simulink model "swingup_student_1"  (R2025b)
settings: Solver=VariableStepAuto  StartTime=0.0  StopTime=30  RelTol=1e-3
undefined symbols (not defined in the file): A, B, C, g, Jp_cm, K, kt, l, mp, mr, r, Rm
libraries: simulink_extras x4, simulink x4
settings Model: Creator=SURESH  LastModifiedBy=USER_NAME
settings RTWCC: GPUComputeCapability=3.5

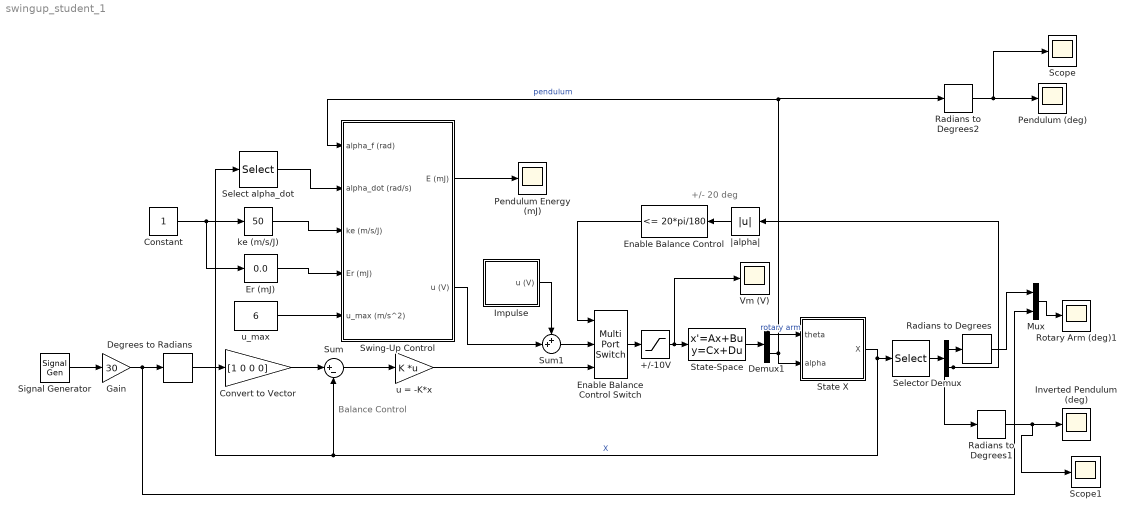
== system swingup_student_1 ==
  note: Balance Control
  note: +/- 20 deg
  +/-10V : Saturate  UpperLimit=10  LowerLimit=-10
  Constant : Constant
  Convert to Vector : Gain  Gain=[1 0 0 0]
  Degrees to Radians : simulink_extras/Transformations/Degrees to Radians
  Demux : Demux  Outputs=2
  Demux1 : Demux  Outputs=2
  Enable Balance Control : simulink/Logic and Bit Operations/Compare To Constant  relop=<=  const=20*pi/180  OutDataTypeStr=uint8  ZeroCross=off
  Enable Balance Control Switch : MultiPortSwitch  DataPortOrder=Zero-based contiguous  Inputs=2  zeroidx=on  SaturateOnIntegerOverflow=off  InputSameDT=off
  Er (mJ) : simulink/Math Operations/Slider Gain  gain=0.0  low=0  high=100
  Gain : Gain  Gain=30
  Impulse : Subsystem
  Inverted Pendulum (deg) : Scope
      settings: ActiveDisplayYMinimum=-5.36133  ActiveDisplayYMaximum=4.30664
  Mux : Mux  Inputs=2
  Pendulum (deg) : Scope
      settings: ActiveDisplayYMinimum=-3.91938  ActiveDisplayYMaximum=3.91995  DataLoggingVariableName=ScopeData2
  Pendulum Energy (mJ) : Scope
      settings: ActiveDisplayYMinimum=30.37049  ActiveDisplayYMaximum=30.37211  DataLoggingVariableName=ScopeData3
  Radians to Degrees : simulink_extras/Transformations/Radians to Degrees
  Radians to Degrees1 : simulink_extras/Transformations/Radians to Degrees
  Radians to Degrees2 : simulink_extras/Transformations/Radians to Degrees
  Rotary Arm (deg)1 : Scope
      settings: ActiveDisplayYMinimum=-42.00725544440256  ActiveDisplayYMaximum=43.502817755714887  DataLoggingVariableName=ScopeData4
  Scope : Scope
      settings: ActiveDisplayYMinimum=-8.16350735550788  ActiveDisplayYMaximum=8.1792601207942344  DataLoggingVariableName=ScopeData5
  Scope1 : Scope
      settings: ActiveDisplayYMinimum=-224.97803  ActiveDisplayYMaximum=224.80225  DataLoggingVariableName=ScopeData6
  Select alpha_dot : Selector  InputPortWidth=4  IndexOptions=Index vector (dialog)  Indices=[4]  OutputSizes=1
  Selector : Selector  InputPortWidth=4  IndexOptions=Index vector (dialog)  Indices=[1 2]  OutputSizes=1
  Signal Generator : SignalGenerator  WaveForm=square  Frequency=0.125
  State X : Subsystem
  State-Space : StateSpace  A=A  B=B  C=C  D=[0;0]  InitialCondition=0
  Sum : Sum  Inputs=|+-
  Sum1 : Sum  Inputs=++|
  Swing-Up Control : Subsystem
  Vm (V) : Scope
      settings: ActiveDisplayYMinimum=-4.30069  ActiveDisplayYMaximum=2.05211
  ke (m/s/J) : simulink/Math Operations/Slider Gain  gain=50  low=0  high=100
  u = -K*x : Gain  Gain=K  Multiplication=Matrix(K*u)
  u_max : Constant  Value=6
  |alpha| : Abs  SaturateOnIntegerOverflow=off
  wires:
  +/-10V/1 -> State-Space/1, Vm (V)/1
  Radians to Degrees/1 -> Mux/1
  Radians to Degrees2/1 -> Scope/1, Pendulum (deg)/1
  Er (mJ)/1 -> Swing-Up Control/4(Er (mJ))
  Convert to Vector/1 -> Sum/1
  Signal Generator/1 -> Gain/1
  Sum1/1 -> Enable Balance Control Switch/2
  Constant/1 -> Er (mJ)/1, ke (m/s/J)/1
  Sum/1 -> u = -K*x/1
  u_max/1 -> Swing-Up Control/5(u_max (m/s^2))
  Gain/1 -> Mux/2, Degrees to Radians/1
  Radians to Degrees1/1 -> Scope1/1, Inverted Pendulum (deg)/1
  Swing-Up Control/1(E (mJ)) -> Pendulum Energy (mJ)/1
  Mux/1 -> Rotary Arm (deg)1/1
  Swing-Up Control/2(u (V)) -> Sum1/2
  Enable Balance Control/1 -> Enable Balance Control Switch/1
  ke (m/s/J)/1 -> Swing-Up Control/3(ke (m/s/J))
  u = -K*x/1 -> Enable Balance Control Switch/3
  Demux/1 -> Radians to Degrees/1
  |alpha|/1 -> Enable Balance Control/1
  Select alpha_dot/1 -> Swing-Up Control/2(alpha_dot (rad/s))
  Degrees to Radians/1 -> Convert to Vector/1
  Enable Balance Control Switch/1 -> +/-10V/1
  Impulse/1(u (V)) -> Sum1/1
  Selector/1 -> Demux/1
  State X/1(X) -> Select alpha_dot/1, Sum/2, Selector/1  "X"
  Demux/2 -> Radians to Degrees1/1, |alpha|/1
  Demux1/1 -> State X/1(theta)  "rotary arm"
  State-Space/1 -> Demux1/1
  Demux1/2 -> Swing-Up Control/1(alpha_f (rad)), Radians to Degrees2/1, State X/2(alpha)  "pendulum"

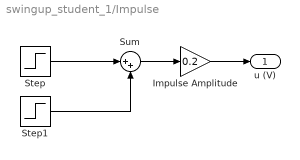
== system swingup_student_1/Impulse ==
  Impulse Amplitude : Gain  Gain=0.2
  Step : Step  SampleTime=0
  Step1 : Step  Time=1.1  After=-1  SampleTime=0
  Sum : Sum  Inputs=|++
  u (V) : Outport
  wires:
  Step1/1 -> Sum/2
  Step/1 -> Sum/1
  Sum/1 -> Impulse Amplitude/1
  Impulse Amplitude/1 -> u (V)/1

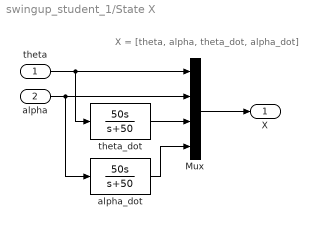
== system swingup_student_1/State X ==
  note: X = [theta, alpha, theta_dot, alpha_dot]
  theta : Inport
  alpha : Inport  Port=2
  Mux : Mux
  alpha_dot : TransferFcn  Numerator=[50 0]  Denominator=[1 50]
  theta_dot : TransferFcn  Numerator=[50 0]  Denominator=[1 50]
  X : Outport  VectorParamsAs1DForOutWhenUnconnected=off
  wires:
  theta_dot/1 -> Mux/3
  alpha_dot/1 -> Mux/4
  alpha/1 -> Mux/2, alpha_dot/1
  Mux/1 -> X/1
  theta/1 -> Mux/1, theta_dot/1

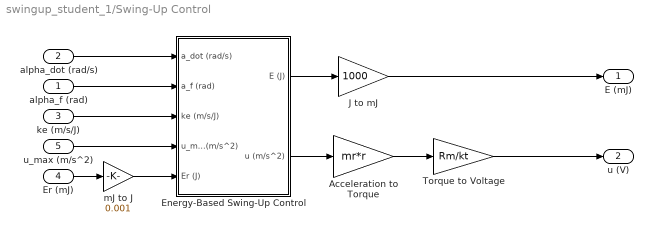
== system swingup_student_1/Swing-Up Control ==
  alpha_f (rad) : Inport
  alpha_dot (rad/s) : Inport  Port=2
  ke (m/s/J) : Inport  Port=3
  Er (mJ) : Inport  Port=4
  u_max (m/s^2) : Inport  Port=5
  Acceleration to Torque : Gain  Gain=mr*r
  Energy-Based Swing-Up Control : Subsystem
  J to mJ : Gain  Gain=1000
  Torque to Voltage : Gain  Gain=Rm/kt
  mJ to J : Gain  Gain=0.001
  E (mJ) : Outport
  u (V) : Outport  Port=2
  wires:
  Energy-Based Swing-Up Control/2(u (m/s^2)) -> Acceleration to Torque/1
  Energy-Based Swing-Up Control/1(E (J)) -> J to mJ/1
  alpha_f (rad)/1 -> Energy-Based Swing-Up Control/2(a_f (rad))
  ke (m/s/J)/1 -> Energy-Based Swing-Up Control/3(ke (m/s/J))
  u_max (m/s^2)/1 -> Energy-Based Swing-Up Control/4(u_max (m/s^2))
  Acceleration to Torque/1 -> Torque to Voltage/1
  Er (mJ)/1 -> mJ to J/1
  J to mJ/1 -> E (mJ)/1
  Torque to Voltage/1 -> u (V)/1
  alpha_dot (rad/s)/1 -> Energy-Based Swing-Up Control/1(a_dot (rad/s))
  mJ to J/1 -> Energy-Based Swing-Up Control/5(Er (J))

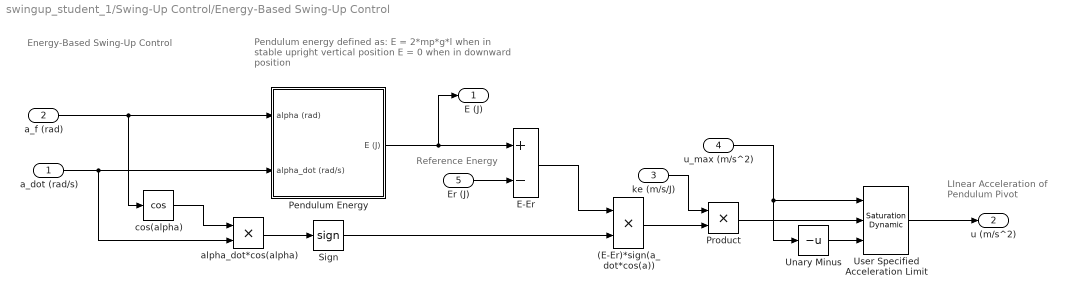
== system swingup_student_1/Swing-Up Control/Energy-Based Swing-Up Control ==
  note: Energy-Based Swing-Up Control
  note: LInear Acceleration of
      | Pendulum Pivot
  note: Reference Energy
  note: Pendulum energy defined as:
      | E = 2*mp*g*l when in stable upright vertical position
      | E = 0 when in downward position
  a_dot (rad/s) : Inport
  a_f (rad) : Inport  Port=2
  ke (m/s/J) : Inport  Port=3
  u_max (m/s^2) : Inport  Port=4
  Er (J) : Inport  Port=5
  (E-Er)*sign(a_dot*cos(a)) : Product  RndMeth=Zero
  E-Er : Sum  Inputs=+-
  Pendulum Energy : Subsystem
  Product : Product  RndMeth=Zero
  Sign : Signum
  Unary Minus : UnaryMinus
  User Specified Acceleration Limit : simulink/Discontinuities/Saturation Dynamic  OutMin=[]  OutMax=[]  OutDataTypeStr=Inherit: Same as second input  OutDataType=fixdt(1, 16)  OutScaling=2^-10  DoSatur=off
  alpha_dot*cos(alpha) : Product  RndMeth=Zero
  cos(alpha) : Trigonometry  Operator=cos
  E (J) : Outport
  u (m/s^2) : Outport  Port=2
  wires:
  a_f (rad)/1 -> Pendulum Energy/1(alpha (rad)), cos(alpha)/1
  Sign/1 -> (E-Er)*sign(a_dot*cos(a))/2
  alpha_dot*cos(alpha)/1 -> Sign/1
  cos(alpha)/1 -> alpha_dot*cos(alpha)/1
  E-Er/1 -> (E-Er)*sign(a_dot*cos(a))/1
  Pendulum Energy/1(E (J)) -> E (J)/1, E-Er/1
  a_dot (rad/s)/1 -> alpha_dot*cos(alpha)/2, Pendulum Energy/2(alpha_dot (rad/s))
  (E-Er)*sign(a_dot*cos(a))/1 -> Product/2
  Er (J)/1 -> E-Er/2
  ke (m/s/J)/1 -> Product/1
  Product/1 -> User Specified Acceleration Limit/2
  u_max (m/s^2)/1 -> User Specified Acceleration Limit/1, Unary Minus/1
  Unary Minus/1 -> User Specified Acceleration Limit/3
  User Specified Acceleration Limit/1 -> u (m/s^2)/1

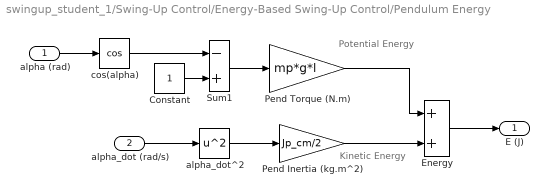
== system swingup_student_1/Swing-Up Control/Energy-Based Swing-Up Control/Pendulum Energy ==
  note: Kinetic Energy
  note: Potential Energy
  alpha (rad) : Inport
  alpha_dot (rad/s) : Inport  Port=2
  Constant : Constant
  Energy : Sum  SaturateOnIntegerOverflow=on
  Pend Inertia (kg.m^2) : Gain  Gain=Jp_cm/2
  Pend Torque (N.m) : Gain  Gain=mp*g*l
  Sum1 : Sum  Inputs=-+  SaturateOnIntegerOverflow=on
  alpha_dot^2 : Math  Operator=square  SignedPower=on
  cos(alpha) : Trigonometry  Operator=cos
  E (J) : Outport
  wires:
  Sum1/1 -> Pend Torque (N.m)/1
  Constant/1 -> Sum1/2
  Pend Inertia (kg.m^2)/1 -> Energy/2
  alpha_dot^2/1 -> Pend Inertia (kg.m^2)/1
  Pend Torque (N.m)/1 -> Energy/1
  alpha (rad)/1 -> cos(alpha)/1
  alpha_dot (rad/s)/1 -> alpha_dot^2/1
  Energy/1 -> E (J)/1
  cos(alpha)/1 -> Sum1/1
